simulink subsystem "Apogee_Delay_Deployment"  (R2024a)
settings: Solver=VariableStepAuto  StartTime=0.0  StopTime=10.0  RelTol=1e-3
undefined symbols (not defined in the file): drogue_apogee_delay
settings Model: Creator=thatf  LastModifiedBy=thatf
settings RTWCC: GPUComputeCapability=3.5

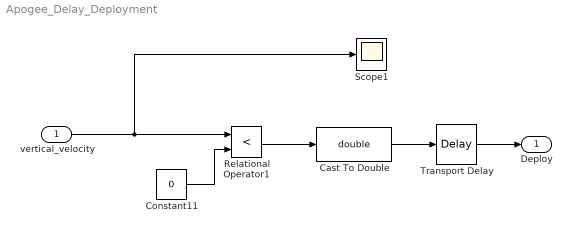
== system Apogee_Delay_Deployment ==
  vertical_velocity : Inport
  Cast To Double : DataTypeConversion  OutDataTypeStr=double  SaturateOnIntegerOverflow=off  RndMeth=Floor
  Constant11 : Constant  Value=0
  Relational Operator1 : RelationalOperator  Operator=<  OutDataTypeStr=boolean  RndMeth=Simplest  InputSameDT=off
  Scope1 : Scope
  Transport Delay : TransportDelay  DelayTime=drogue_apogee_delay
  Deploy : Outport
  wires:
  Transport Delay/1 -> Deploy/1
  vertical_velocity/1 -> Relational Operator1/1, Scope1/1
  Constant11/1 -> Relational Operator1/2
  Relational Operator1/1 -> Cast To Double/1
  Cast To Double/1 -> Transport Delay/1
